simulink model "shower"  (R2018b)
settings: Solver=VariableStepAuto  StartTime=0.0  StopTime=10.0  RelTol=1e-3  EnableMultiTasking=on
libraries: fuzblock x1
settings Model: Creator=Ranish  LastModifiedBy=Ranish
settings DataIOCC: LimitDataPoints=on
settings OptimizationCC: LifeSpan=inf
settings DebuggingCC: AllowSymbolicDim=off  SFUnexpectedBacktrackingDiag=warning  SFNoUnconditionalDefaultTransitionDiag=warning  SFExecutionAtInitializationDiag=none
settings SFSimCC: SimUseLocalCustomCode=off
settings RTWCC: RTWUseLocalCustomCode=off
settings CodeAppCC: StateflowObjectComments=on
settings GRTTargetCC: TargetLangStandard=C89/C90 (ANSI)  GeneratePreprocessorConditionals=Disable all
settings ConfigComp: CovMetricSettings=dw  CovHtmlReporting=on  CovSaveCumulativeToWorkspaceVar=on  CovSaveSingleToWorkspaceVar=on  CovExternalEMLEnable=off  CovSFcnEnable=off
settings SimscapeCC: SimscapeNominalValues="[{\"value\":\"10\",\"unit\":\"V\"},{\"value\":\"1\",\"unit\":\"A\"},{\"value\":\"10\",\"unit\":\"N*m\"},{\"value\":\"10\",\"unit\":\"bar\"},{\"value\":\"100\",\"unit\":\"kJ/kg\"},{\"value\":\"1\",\"unit\":\"kW\"},{\"value\":\"300\",\"unit\":\"K\"},{\"value\":\"100\",\"unit\":\"cm^3/s\"},{\"value\":\"1\",\"unit\":\"kN\"},{\"value\":\"1\",\"unit\":\"g/cm^3\"},{\"value\":\"1\",\"unit\":\"l\"},{\"value\":\"1\",\"unit\":\"cm^2\"},{\"value\":\"60\",\"unit\":\"Hz\"}]"  SimscapeLogType=all  SimscapeLogDataHistory=10000
settings ConfigurationSet: Description=SimMechanics 2G

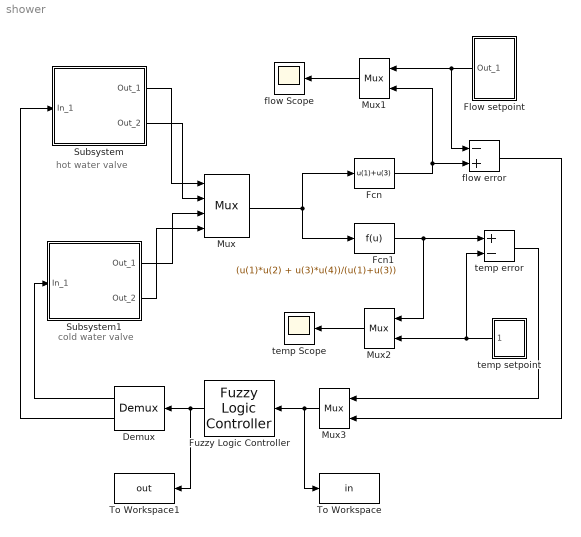
== system shower ==
  note: cold water valve
  note: hot water valve
  Demux : Demux  Outputs=2
  Fcn : Fcn  Expr=u(1)+u(3)
  Fcn1 : Fcn  Expr=(u(1)*u(2) + u(3)*u(4))/(u(1)+u(3))
  "Flow setpoint " : Subsystem
  Fuzzy Logic Controller : fuzblock/Fuzzy Logic  Controller  FIS=controller.FIS  OutputSampleNumber=101  DataType=double  FuzzifiedInputs=off  RuleFiringStrengths=off  RuleOutputs=off  AggregatedOutputs=off  SimulateUsing=Interpreted execution  OutOfRangeInputValueMessage=warning  NoRuleFiredMessage=warning  EmptyOutputFuzzySetMessage=warning
  Mux : Mux
  Mux1 : Mux  Inputs=2
  Mux2 : Mux  Inputs=2
  Mux3 : Mux  Inputs=2
  Subsystem : Subsystem
  Subsystem1 : Subsystem
  To Workspace : ToWorkspace  VariableName=in
  To Workspace1 : ToWorkspace  VariableName=out
  flow Scope : Scope
  "flow error " : Sum  Inputs=-+
  temp Scope : Scope
  "temp setpoint " : Subsystem
  "temp error " : Sum  Inputs=+-
  wires:
  Subsystem/2(Out_2) -> Mux/2
  Subsystem/1(Out_1) -> Mux/1
  Subsystem1/1(Out_1) -> Mux/3
  Subsystem1/2(Out_2) -> Mux/4
  Mux/1 -> Fcn/1, Fcn1/1
  "Flow setpoint "/1(Out_1) -> "flow error "/1, Mux1/1
  "temp setpoint "/1(Out_1) -> Mux2/2, "temp error "/2
  Mux1/1 -> flow Scope/1
  Fcn/1 -> Mux1/2, "flow error "/2
  Fcn1/1 -> Mux2/1, "temp error "/1
  Mux3/1 -> To Workspace/1, Fuzzy Logic Controller/1
  "temp error "/1 -> Mux3/1
  "flow error "/1 -> Mux3/2
  Fuzzy Logic Controller/1 -> To Workspace1/1, Demux/1
  Demux/1 -> Subsystem1/1(In_1)
  Demux/2 -> Subsystem/1(In_1)
  Mux2/1 -> temp Scope/1

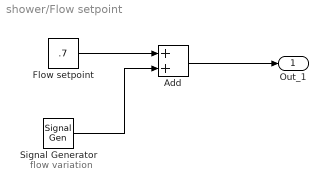
== system shower/Flow setpoint  ==
  note: flow variation
  Add : Sum
  "Flow setpoint " : Constant  Value=.7
  Signal Generator : SignalGenerator  WaveForm=square  Amplitude=0.200000  Frequency=0.300000  Units=rad/sec
  Out_1 : Outport
  wires:
  Signal Generator/1 -> Add/2
  "Flow setpoint "/1 -> Add/1
  Add/1 -> Out_1/1

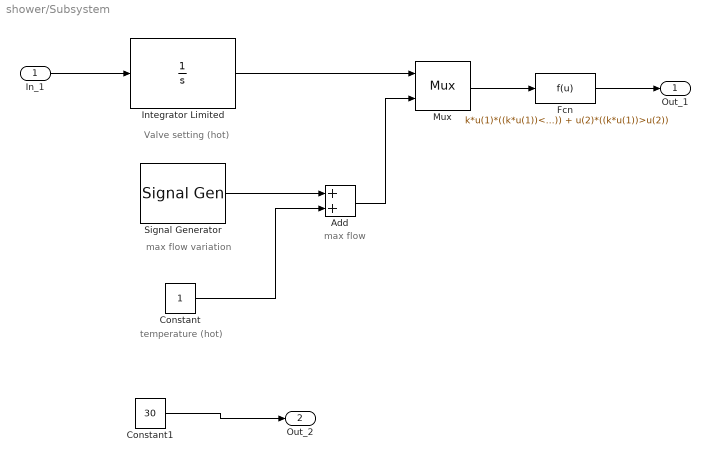
== system shower/Subsystem ==
  note: max flow
  note: temperature (hot)
  note: max flow variation
  note: Valve setting (hot)
  In_1 : Inport
  Add : Sum
  Constant : Constant
  Constant1 : Constant  Value=30
  Fcn : Fcn  Expr=k*u(1)*((k*u(1))<=u(2)) + u(2)*((k*u(1))>u(2))
  Integrator Limited : Integrator  InitialCondition=0.1  LimitOutput=on  UpperSaturationLimit=2  LowerSaturationLimit=0.001
      mask Display: plot(-1,-0.2,3.5,1.2,[0.05,1,2,2.9],[0,0,1,1]);disp(' 1/s    ')
  Mux : Mux  Inputs=2
  Signal Generator : SignalGenerator  Amplitude=0.000000  Frequency=0.300000  Units=rad/sec
  Out_1 : Outport
  Out_2 : Outport  Port=2
  wires:
  Constant1/1 -> Out_2/1
  In_1/1 -> Integrator Limited/1
  Integrator Limited/1 -> Mux/1
  Signal Generator/1 -> Add/1
  Constant/1 -> Add/2
  Add/1 -> Mux/2
  Mux/1 -> Fcn/1
  Fcn/1 -> Out_1/1

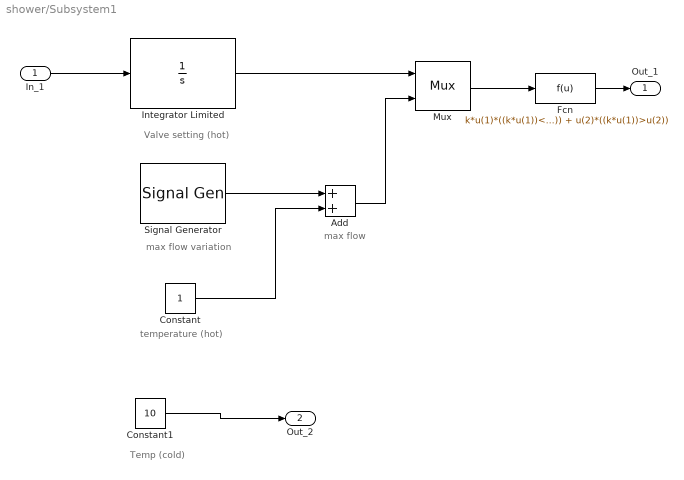
== system shower/Subsystem1 ==
  note: Temp (cold)
  note: Valve setting (hot)
  note: max flow variation
  note: temperature (hot)
  note: max flow
  In_1 : Inport
  Add : Sum
  Constant : Constant
  Constant1 : Constant  Value=10
  Fcn : Fcn  Expr=k*u(1)*((k*u(1))<=u(2)) + u(2)*((k*u(1))>u(2))
  Integrator Limited : Integrator  InitialCondition=0.1  LimitOutput=on  UpperSaturationLimit=2  LowerSaturationLimit=0.001
      mask Display: plot(-1,-0.2,3.5,1.2,[0.05,1,2,2.9],[0,0,1,1]);disp(' 1/s    ')
  Mux : Mux  Inputs=2
  Signal Generator : SignalGenerator  Amplitude=0.000000  Frequency=0.101325  Units=rad/sec
  Out_1 : Outport
  Out_2 : Outport  Port=2
  wires:
  Mux/1 -> Fcn/1
  Add/1 -> Mux/2
  Constant/1 -> Add/2
  Signal Generator/1 -> Add/1
  Integrator Limited/1 -> Mux/1
  In_1/1 -> Integrator Limited/1
  Constant1/1 -> Out_2/1
  Fcn/1 -> Out_1/1

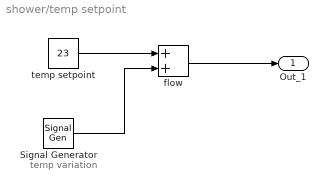
== system shower/temp setpoint  ==
  note: temp variation
  Signal Generator : SignalGenerator  WaveForm=square  Amplitude=4.000000  Frequency=0.214320  Units=rad/sec
  flow : Sum
  "temp setpoint " : Constant  Value=23
  Out_1 : Outport
  wires:
  flow/1 -> Out_1/1
  "temp setpoint "/1 -> flow/1
  Signal Generator/1 -> flow/2
